simulink model "PMSM_Sinusoidal_Drive"  (Simulink 7.8)
settings: Solver=FixedStepDiscrete  StartTime=0.0  StopTime=10.0  FixedStep=.0001  RelTol=1e-3
undefined symbols (not defined in the file): abc, alphabeta, dq, MicrochipMotorControlTools, to
settings Model: Creator=Marx  LastModifiedBy=Pavlo
settings OptimizationCC: OptimizeModelRefInitCode=on  LifeSpan=1
settings HardwareCC: ProdBitPerInt=16  ProdBitPerPointer=16  ProdIntDivRoundTo=Zero  ProdEndianess=LittleEndian  ProdWordSize=16  ProdHWDeviceType=Microchip->dsPIC
settings RTWCC: SystemTargetFile=ert.tlc  GenCodeOnly=on  TemplateMakefile=ert_default_tmf  Description=Embedded Coder  ProcessScript=ert_make_rtw_hook  RTWCompilerOptimization=On
settings CodeAppCC: IgnoreCustomStorageClasses=off
settings ERTTargetCC: MultiwordLength=2048  GenerateSampleERTMain=on  ERTCustomFileTemplate=example_file_process.tlc  ConvertIfToSwitch=off  SuppressUnreachableDefaultCases=off
settings SimEventsCC: propDiagStatOutput=1

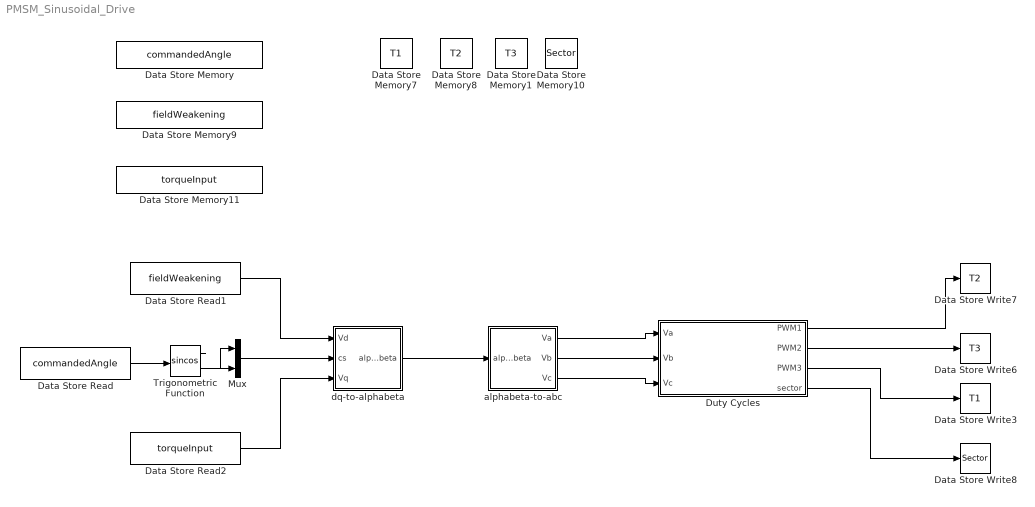
== system PMSM_Sinusoidal_Drive ==
  Data Store Memory : DataStoreMemory  DataStoreName=commandedAngle  ReadBeforeWriteMsg=warning  WriteAfterWriteMsg=warning  WriteAfterReadMsg=warning  OutDataTypeStr=single
      settings: RTWStateStorageClass=ExportedGlobal
  Data Store Memory1 : DataStoreMemory  DataStoreName=T3  ReadBeforeWriteMsg=warning  WriteAfterWriteMsg=warning  WriteAfterReadMsg=warning  OutDataTypeStr=single
  Data Store Memory10 : DataStoreMemory  DataStoreName=Sector  ReadBeforeWriteMsg=warning  WriteAfterWriteMsg=warning  WriteAfterReadMsg=warning  OutDataTypeStr=single
  Data Store Memory11 : DataStoreMemory  DataStoreName=torqueInput  ReadBeforeWriteMsg=warning  WriteAfterWriteMsg=warning  WriteAfterReadMsg=warning  OutDataTypeStr=single
      settings: RTWStateStorageClass=ExportedGlobal
  Data Store Memory7 : DataStoreMemory  DataStoreName=T1  ReadBeforeWriteMsg=warning  WriteAfterWriteMsg=warning  WriteAfterReadMsg=warning  OutDataTypeStr=single
  Data Store Memory8 : DataStoreMemory  DataStoreName=T2  ReadBeforeWriteMsg=warning  WriteAfterWriteMsg=warning  WriteAfterReadMsg=warning  OutDataTypeStr=single
  Data Store Memory9 : DataStoreMemory  DataStoreName=fieldWeakening  ReadBeforeWriteMsg=warning  WriteAfterWriteMsg=warning  WriteAfterReadMsg=warning  OutDataTypeStr=single
      settings: RTWStateStorageClass=ExportedGlobal
  Data Store Read : DataStoreRead  DataStoreName=commandedAngle
  Data Store Read1 : DataStoreRead  DataStoreName=fieldWeakening
  Data Store Read2 : DataStoreRead  DataStoreName=torqueInput
  Data Store Write3 : DataStoreWrite  DataStoreName=T1
  Data Store Write6 : DataStoreWrite  DataStoreName=T3
  Data Store Write7 : DataStoreWrite  DataStoreName=T2
  Data Store Write8 : DataStoreWrite  DataStoreName=Sector
  Duty Cycles : MATLAB Function  TreatAsAtomicUnit=on
  Mux : Mux  Inputs=2
  Trigonometric Function : Trigonometry  Operator=sincos
  alphabeta-to-abc : Subsystem  AncestorBlock=MicrochipMotorControlTools/alphabeta-to-abc
  dq-to-alphabeta : Subsystem  AncestorBlock=MicrochipMotorControlTools/dq-to-alphabeta
  wires:
  Mux/1 -> dq-to-alphabeta/2(cs)
  dq-to-alphabeta/1(alphabeta) -> alphabeta-to-abc/1(alphabeta)
  alphabeta-to-abc/1(Va) -> Duty Cycles/1(Va)
  alphabeta-to-abc/2(Vb) -> Duty Cycles/2(Vb)
  alphabeta-to-abc/3(Vc) -> Duty Cycles/3(Vc)
  Data Store Read1/1 -> dq-to-alphabeta/1(Vd)
  Data Store Read2/1 -> dq-to-alphabeta/3(Vq)
  Data Store Read/1 -> Trigonometric Function/1
  Duty Cycles/1(PWM1) -> Data Store Write7/1
  Duty Cycles/2(PWM2) -> Data Store Write6/1
  Duty Cycles/3(PWM3) -> Data Store Write3/1
  Duty Cycles/4(sector) -> Data Store Write8/1
  Trigonometric Function/2 -> Mux/1
  Trigonometric Function/1 -> Mux/2

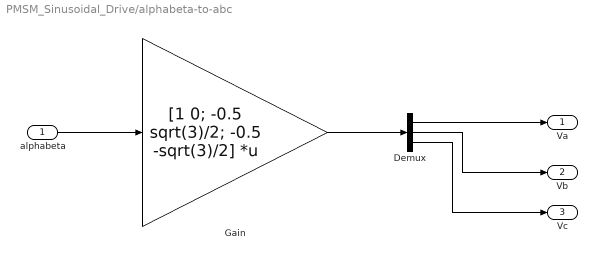
== system PMSM_Sinusoidal_Drive/alphabeta-to-abc ==
  alphabeta : Inport
  Demux : Demux  Outputs=3
  Gain : Gain  Gain=[1 0; -0.5 sqrt(3)/2; -0.5 -sqrt(3)/2]  Multiplication=Matrix(K*u)  OutDataTypeStr=single
  Va : Outport  OutDataTypeStr=single
  Vb : Outport  Port=2  OutDataTypeStr=single
  Vc : Outport  Port=3  OutDataTypeStr=single
  wires:
  alphabeta/1 -> Gain/1
  Gain/1 -> Demux/1
  Demux/1 -> Va/1
  Demux/2 -> Vb/1
  Demux/3 -> Vc/1

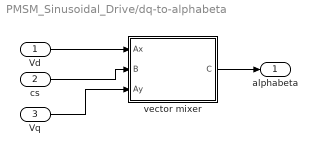
== system PMSM_Sinusoidal_Drive/dq-to-alphabeta ==
  Vd : Inport
  cs : Inport  Port=2
  Vq : Inport  Port=3
  vector mixer : Subsystem  AncestorBlock=MicrochipMotorControlTools/vector mixer
  alphabeta : Outport
  wires:
  cs/1 -> vector mixer/2(B)
  Vd/1 -> vector mixer/1(Ax)
  vector mixer/1(C) -> alphabeta/1
  Vq/1 -> vector mixer/3(Ay)

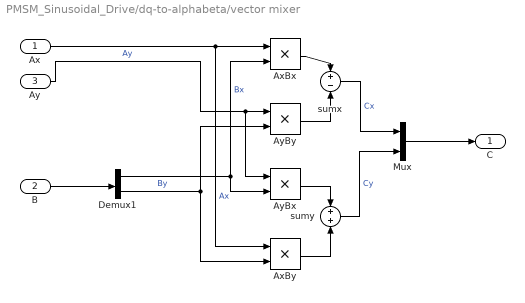
== system PMSM_Sinusoidal_Drive/dq-to-alphabeta/vector mixer ==
  Ax : Inport
  B : Inport  Port=2
  Ay : Inport  Port=3
  AxBx : Product  RndMeth=Zero  OutDataTypeStr=Inherit: Same as first input
  AxBy : Product  RndMeth=Zero  OutDataTypeStr=Inherit: Same as first input
  AyBx : Product  RndMeth=Zero  OutDataTypeStr=Inherit: Same as first input
  AyBy : Product  RndMeth=Zero  OutDataTypeStr=Inherit: Same as first input
  Demux1 : Demux  Outputs=2
  Mux : Mux  Inputs=2
  sumx : Sum  Inputs=+|-
  sumy : Sum  Inputs=+|+
  C : Outport
  wires:
  sumx/1 -> Mux/1  "Cx"
  B/1 -> Demux1/1
  Demux1/1 -> AyBx/2, AxBx/2  "Bx"
  Demux1/2 -> AxBy/2, AyBy/2  "By"
  sumy/1 -> Mux/2  "Cy"
  AxBy/1 -> sumy/2
  AyBx/1 -> sumy/1
  AxBx/1 -> sumx/1
  AyBy/1 -> sumx/2
  Ay/1 -> AyBy/1, AyBx/1  "Ay"
  Ax/1 -> AxBy/1, AxBx/1  "Ax"
  Mux/1 -> C/1

== matlab function Duty Cycles ==
  data: PWM1 output single; Va input single; PWM2 output single; PWM3 output single; sector output double; Vb input double; Vc input double
function [PWM1, PWM2, PWM3, sector]  = DutyCycleCalc(Va, Vb, Vc)
%#codegen
PWM = single(100);

Ta = single(0);

if (Va >= 0)
    if (Vb >= 0)
        %Sector 3, 0 - 60 Degrees
        T1 = Vb;
        T2 = Va;
    
        T1 = T1*PWM;
        T2 = T2*PWM;
        Tc = (PWM-T1-T2)/2;
        Tb = Ta + T1;
        Ta = Tb + T2;
    
        PWM1 = single(0);
        PWM2 = Tb;
        PWM3 = Ta;
        sector = single(3);
    else
        if (Vc >= 0)
           %Sector 5, 120 - 180 Degrees
            T1 = Va;
            T2 = Vc;
    
            T1 = T1*PWM;
            T2 = T2*PWM;
            Tc = (PWM-T1-T2)/2;
            Tb = Ta + T1;
            Ta = Tb + T2;
    
            PWM1 = Ta;
            PWM2 = single(0);
            PWM3 = Tb;
            sector = single(5);
        else
            %Sector 1, 60 - 120 Degrees
            T1 = -Vb;
            T2 = -Vc;
    
            T1 = T1*PWM;
            T2 = T2*PWM;
            Tc = (PWM-T1-T2)/2;
            Tb = Ta + T1;
            Ta = Tb + T2;
    
            PWM1 = Tb;
            PWM2 = single(0);
            PWM3 = Ta;
            sector = single(1);
        end
    end
else
    if (Vb >= 0)
        if (Vc >= 0)
            %Sector 6, 240 - 300 Degrees
            T1 = Vc;
            T2 = Vb;
    
            T1 = T1*PWM;
            T2 = T2*PWM;
            Tc = (PWM-T1-T2)/2;
            Tb = Ta + T1;
            Ta = Tb + T2;
    
            PWM1 = Tb;
            PWM2 = Ta;
            PWM3 = single(0);
            sector = single(6);
        else
            %Sector 2, 300 - 0 Degrees
            T1 = -Vc;
            T2 = -Va;
    
            T1 = T1*PWM;
            T2 = T2*PWM;
            Tc = (PWM-T1-T2)/2;
            Tb = Ta + T1;
            Ta = Tb + T2;
    
            PWM1 = single(0);
            PWM2 = Ta;
            PWM3 = Tb;
            sector = single(2);
        end
    else
        %Sector 4, 180 - 240 Degrees
        T1 = -Va;
        T2 = -Vb;
    
        T1 = T1*PWM;
        T2 = T2*PWM;
        Tc = (PWM-T1-T2)/2;
        Tb = Ta + T1;
        Ta = Tb + T2;
    
        PWM1 = Ta;
        PWM2 = Tb;
        PWM3 = single(0);
        sector = single(4);
    end
end

end
